simulink model "L15SimMSD"  (R2020a)
settings: Solver=FixedStepAuto  StartTime=0.0  StopTime=100.0  FixedStep=0.01  RelTol=1e-3
InitFcn:
  | ParametersMSD;
values from neighbouring files (symbols this model uses):
  A = [0 1 ; -k/m -b/m]    [L15ParametersMSD.m]
  B = [0 ; 1/m]    [L15ParametersMSD.m]
  K = [k1 k2]    [L15ParametersMSD.m]
  x0 = [p0 ; v0]    [L15ParametersMSD.m]
settings Model: Creator=vcichella  LastModifiedBy=vcichella

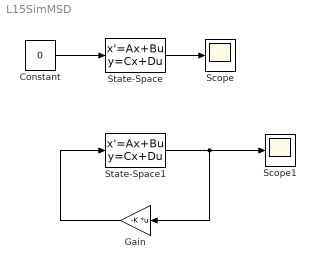
== system L15SimMSD ==
  Constant : Constant  Value=0
  Gain : Gain  Gain=-K  Multiplication=Matrix(K*u)
  Scope : Scope
  Scope1 : Scope
  State-Space : StateSpace  A=A  B=B  C=eye(2)  D=zeros(2,1)  InitialCondition=x0
  State-Space1 : StateSpace  A=A  B=B  C=eye(2)  D=zeros(2,1)  InitialCondition=x0
  wires:
  Constant/1 -> State-Space/1
  State-Space/1 -> Scope/1
  State-Space1/1 -> Scope1/1, Gain/1
  Gain/1 -> State-Space1/1
